simulink model "Lateral_control_of_HST"  (R2023b)
settings: Solver=ode45  StartTime=0.0  StopTime=100  FixedStep=0.001  RelTol=1e-3
InitFcn:
  | Parameters_and_initial_conditions;
values from neighbouring files (symbols this model uses):
  A_a = 2.119e-7    (= 2.119e-07)    [Parameters_and_initial_conditions.m]
  A_v = 4.032e-7    (= 4.032e-07)    [Parameters_and_initial_conditions.m]
  b = 0.7465    [Parameters_and_initial_conditions.m]
  c_px = 0    [Parameters_and_initial_conditions.m]
  c_py = 0    [Parameters_and_initial_conditions.m]
  c_pz = 1.5e4    (= 15000)    [Parameters_and_initial_conditions.m]
  c_sx = 0    [Parameters_and_initial_conditions.m]
  c_sy = 2e4    (= 20000)    [Parameters_and_initial_conditions.m]
  c_sz = 8e4    (= 80000)    [Parameters_and_initial_conditions.m]
  d_p = 1    [Parameters_and_initial_conditions.m]
  d_s = 1    [Parameters_and_initial_conditions.m]
  f_11 = 1.12e7    (= 11200000)    [Parameters_and_initial_conditions.m]
  f_22 = 9.98e6    (= 9980000)    [Parameters_and_initial_conditions.m]
  h_cs = 0.98    [Parameters_and_initial_conditions.m]
  h_ts = 0.0945    [Parameters_and_initial_conditions.m]
  h_tw = 0.1745    [Parameters_and_initial_conditions.m]
  J_cx = 89396    [Parameters_and_initial_conditions.m]
  J_cz = 2485756    [Parameters_and_initial_conditions.m]
  J_tx = 2650    [Parameters_and_initial_conditions.m]
  J_tz = 3000    [Parameters_and_initial_conditions.m]
  J_wz = 1200    [Parameters_and_initial_conditions.m]
  k11 = 1.88e7    (= 18800000)    [Parameters_and_initial_conditions.m]
  k12 = 5.807e5    (= 580700)    [Parameters_and_initial_conditions.m]
  k13 = 3.68e6    (= 3680000)    [Parameters_and_initial_conditions.m]
  k14 = 2.64e1    (= 26.4)    [Parameters_and_initial_conditions.m]
  k21 = 1.88e7    (= 18800000)    [Parameters_and_initial_conditions.m]
  k22 = 5.807e5    (= 580700)    [Parameters_and_initial_conditions.m]
  k23 = 3.68e6    (= 3680000)    [Parameters_and_initial_conditions.m]
  k24 = 2.64e1    (= 26.4)    [Parameters_and_initial_conditions.m]
  K_gpsi = -7834    [Parameters_and_initial_conditions.m]
  K_gy = 5014    [Parameters_and_initial_conditions.m]
  k_px = 1.45e7    (= 14500000)    [Parameters_and_initial_conditions.m]
  k_py = 7.5e6    (= 7500000)    [Parameters_and_initial_conditions.m]
  k_pz = 6.65e5    (= 665000)    [Parameters_and_initial_conditions.m]
  k_sx = 2.08e5    (= 208000)    [Parameters_and_initial_conditions.m]
  k_sy = 2.08e5    (= 208000)    [Parameters_and_initial_conditions.m]
  k_sz = 3.5e5    (= 350000)    [Parameters_and_initial_conditions.m]
  kd = 1    [Parameters_and_initial_conditions.m]
  kp = 3    [Parameters_and_initial_conditions.m]
  l = 9    [Parameters_and_initial_conditions.m]
  l_t = 1.25    [Parameters_and_initial_conditions.m]
  Lambda_a = 6.125e-7    (= 6.125e-07)    [Parameters_and_initial_conditions.m]
  lambda_e = 0.05    [Parameters_and_initial_conditions.m]
  Lambda_v = 1.08e-6    (= 1.08e-06)    [Parameters_and_initial_conditions.m]
  m_c = 40000    [Parameters_and_initial_conditions.m]
  m_t = 2280    [Parameters_and_initial_conditions.m]
  m_w = 1650    [Parameters_and_initial_conditions.m]
  Omega_c = 0.8246    [Parameters_and_initial_conditions.m]
  Omega_r = 0.0206    [Parameters_and_initial_conditions.m]
  Omega_s = 0.438    [Parameters_and_initial_conditions.m]
  psi_c_dot_initial = 0    [Parameters_and_initial_conditions.m]
  psi_c_initial = 0    [Parameters_and_initial_conditions.m]
  psi_t1_dot_initial = 0    [Parameters_and_initial_conditions.m]
  psi_t1_initial = 0    [Parameters_and_initial_conditions.m]
  psi_t2_dot_initial = 0    [Parameters_and_initial_conditions.m]
  psi_t2_initial = 0    [Parameters_and_initial_conditions.m]
  psi_w1_dot_initial = 0    [Parameters_and_initial_conditions.m]
  psi_w1_initial = 0    [Parameters_and_initial_conditions.m]
  psi_w2_dot_initial = 0    [Parameters_and_initial_conditions.m]
  psi_w2_initial = 0    [Parameters_and_initial_conditions.m]
  psi_w3_dot_initial = 0    [Parameters_and_initial_conditions.m]
  psi_w3_initial = 0    [Parameters_and_initial_conditions.m]
  psi_w4_dot_initial = 0    [Parameters_and_initial_conditions.m]
  psi_w4_initial = 0    [Parameters_and_initial_conditions.m]
  r_0 = 0.4575    [Parameters_and_initial_conditions.m]
  sigma = 0.05    [Parameters_and_initial_conditions.m]
  T1 = 0.15    [Parameters_and_initial_conditions.m]
  T2 = 0.04    [Parameters_and_initial_conditions.m]
  Tff = 0.1*tau    (= 0.3)    [Parameters_and_initial_conditions.m]
  Tff2 = 0.2*tau    (= 0.6)    [Parameters_and_initial_conditions.m]
  theta_c_dot_initial = 0    [Parameters_and_initial_conditions.m]
  theta_c_initial = 0    [Parameters_and_initial_conditions.m]
  theta_t1_dot_initial = 0    [Parameters_and_initial_conditions.m]
  theta_t1_initial = 0    [Parameters_and_initial_conditions.m]
  theta_t2_dot_initial = 0    [Parameters_and_initial_conditions.m]
  theta_t2_initial = 0    [Parameters_and_initial_conditions.m]
  Tnn = 0.5*tau    (= 1.5)    [Parameters_and_initial_conditions.m]
  Tnn2 = 1*tau    (= 3)    [Parameters_and_initial_conditions.m]
  V = 75    [Parameters_and_initial_conditions.m]
  y_c_dot_initial = 0    [Parameters_and_initial_conditions.m]
  y_c_initial = 0    [Parameters_and_initial_conditions.m]
  y_t1_dot_initial = 0    [Parameters_and_initial_conditions.m]
  y_t1_initial = 0    [Parameters_and_initial_conditions.m]
  y_t2_dot_initial = 0    [Parameters_and_initial_conditions.m]
  y_t2_initial = 0    [Parameters_and_initial_conditions.m]
  y_w1_dot_initial = 0    [Parameters_and_initial_conditions.m]
  y_w1_initial = 0    [Parameters_and_initial_conditions.m]
  y_w2_dot_initial = 0    [Parameters_and_initial_conditions.m]
  y_w2_initial = 0    [Parameters_and_initial_conditions.m]
  y_w3_dot_initial = 0    [Parameters_and_initial_conditions.m]
  y_w3_initial = 0    [Parameters_and_initial_conditions.m]
  y_w4_dot_initial = 0    [Parameters_and_initial_conditions.m]
  y_w4_initial = 0    [Parameters_and_initial_conditions.m]
libraries: simulink x6, dspsrcs4 x1
(part 2 of 2)

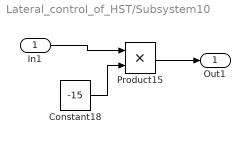
== system Lateral_control_of_HST/Subsystem10 ==
  In1 : Inport
  Constant18 : Constant  Value=-15
  Product15 : Product
  Out1 : Outport
  wires:
  Constant18/1 -> Product15/2
  In1/1 -> Product15/1
  Product15/1 -> Out1/1

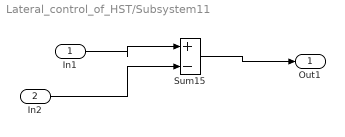
== system Lateral_control_of_HST/Subsystem11 ==
  In1 : Inport
  In2 : Inport  Port=2
  Sum15 : Sum  Inputs=|+-
  Out1 : Outport
  wires:
  In2/1 -> Sum15/2
  In1/1 -> Sum15/1
  Sum15/1 -> Out1/1

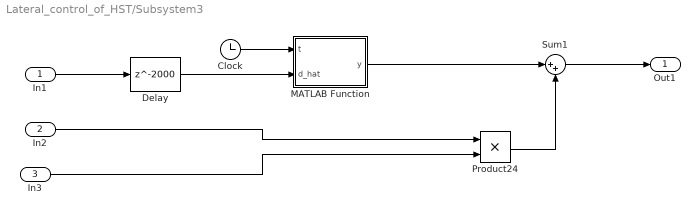
== system Lateral_control_of_HST/Subsystem3 ==
  In1 : Inport
  In2 : Inport  Port=2
  In3 : Inport  Port=3
  Clock : Clock
  Delay : Delay  DelayLength=2000
  MATLAB Function : MATLAB Function  TreatAsAtomicUnit=on
  Product24 : Product
  Sum1 : Sum  Inputs=|++
  Out1 : Outport
  wires:
  Clock/1 -> MATLAB Function/1(t)
  Product24/1 -> Sum1/2
  Sum1/1 -> Out1/1
  In2/1 -> Product24/1
  MATLAB Function/1(y) -> Sum1/1
  Delay/1 -> MATLAB Function/2(d_hat)
  In1/1 -> Delay/1
  In3/1 -> Product24/2

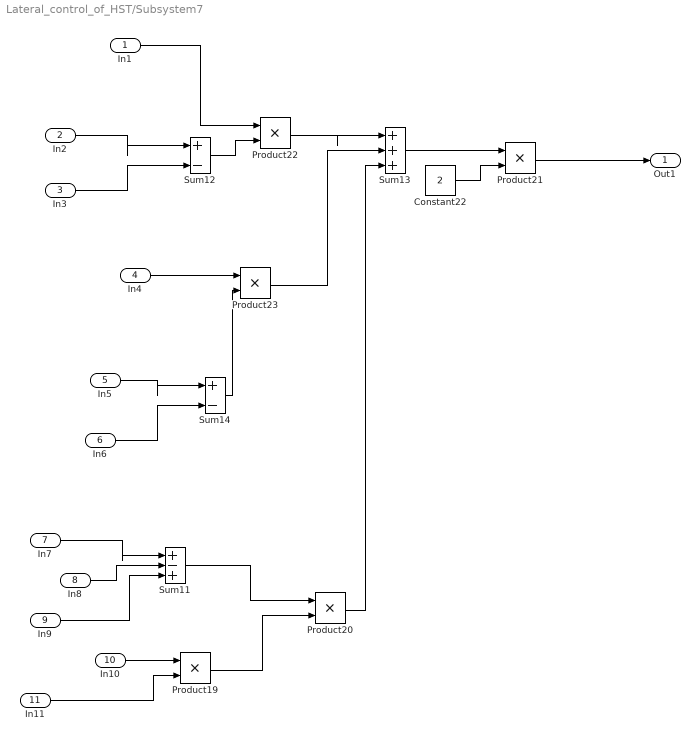
== system Lateral_control_of_HST/Subsystem7 ==
  In1 : Inport
  In2 : Inport  Port=2
  In3 : Inport  Port=3
  In4 : Inport  Port=4
  In5 : Inport  Port=5
  In6 : Inport  Port=6
  In7 : Inport  Port=7
  In8 : Inport  Port=8
  In9 : Inport  Port=9
  In10 : Inport  Port=10
  In11 : Inport  Port=11
  Constant22 : Constant  Value=2
  Product{19..23} (5 alike) : Product
  Sum11 : Sum  Inputs=|+-+
  Sum12 : Sum  Inputs=|+-
  Sum13 : Sum  Inputs=|+++
  Sum14 : Sum  Inputs=|+-
  Out1 : Outport
  wires:
  Product22/1 -> Sum13/1
  In5/1 -> Sum14/1
  Sum13/1 -> Product21/1
  In6/1 -> Sum14/2
  Sum11/1 -> Product20/1
  Product19/1 -> Product20/2
  Sum14/1 -> Product23/2
  In7/1 -> Sum11/1
  Product23/1 -> Sum13/2
  Sum12/1 -> Product22/2
  In2/1 -> Sum12/1
  Product20/1 -> Sum13/3
  Constant22/1 -> Product21/2
  In10/1 -> Product19/1
  In9/1 -> Sum11/3
  In4/1 -> Product23/1
  In3/1 -> Sum12/2
  In1/1 -> Product22/1
  Product21/1 -> Out1/1
  In11/1 -> Product19/2
  In8/1 -> Sum11/2

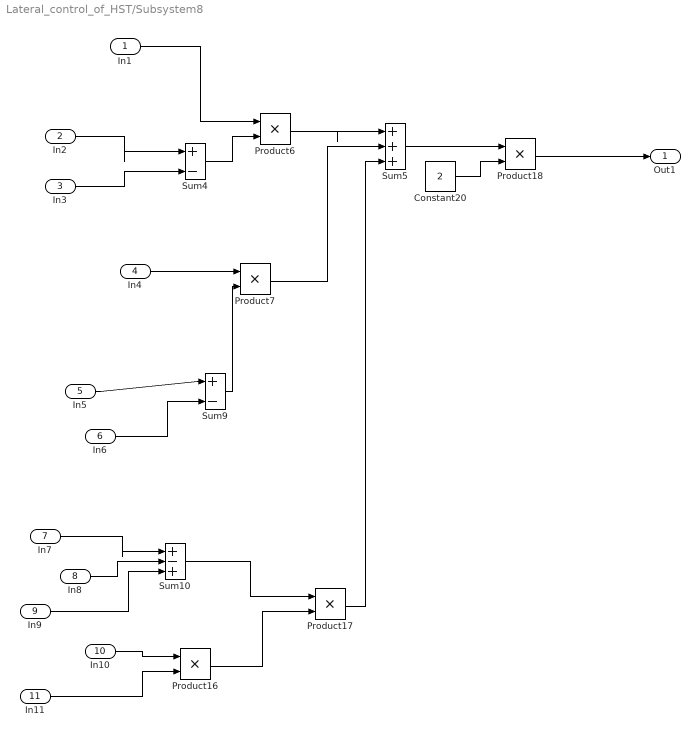
== system Lateral_control_of_HST/Subsystem8 ==
  In1 : Inport
  In2 : Inport  Port=2
  In3 : Inport  Port=3
  In4 : Inport  Port=4
  In5 : Inport  Port=5
  In6 : Inport  Port=6
  In7 : Inport  Port=7
  In8 : Inport  Port=8
  In9 : Inport  Port=9
  In10 : Inport  Port=10
  In11 : Inport  Port=11
  Constant20 : Constant  Value=2
  Product{6..7,16..18} (5 alike) : Product
  Sum10 : Sum  Inputs=|+-+
  Sum4 : Sum  Inputs=|+-
  Sum5 : Sum  Inputs=|+++
  Sum9 : Sum  Inputs=|+-
  Out1 : Outport
  wires:
  Constant20/1 -> Product18/2
  Product6/1 -> Sum5/1
  Sum9/1 -> Product7/2
  Product17/1 -> Sum5/3
  Sum4/1 -> Product6/2
  In6/1 -> Sum9/2
  Product16/1 -> Product17/2
  Sum5/1 -> Product18/1
  In9/1 -> Sum10/3
  Product7/1 -> Sum5/2
  In1/1 -> Product6/1
  Sum10/1 -> Product17/1
  Product18/1 -> Out1/1
  In8/1 -> Sum10/2
  In4/1 -> Product7/1
  In5/1 -> Sum9/1
  In7/1 -> Sum10/1
  In3/1 -> Sum4/2
  In2/1 -> Sum4/1
  In11/1 -> Product16/2
  In10/1 -> Product16/1

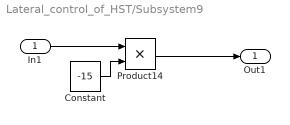
== system Lateral_control_of_HST/Subsystem9 ==
  In1 : Inport
  Constant : Constant  Value=-15
  Product14 : Product
  Out1 : Outport
  wires:
  Constant/1 -> Product14/2
  In1/1 -> Product14/1
  Product14/1 -> Out1/1

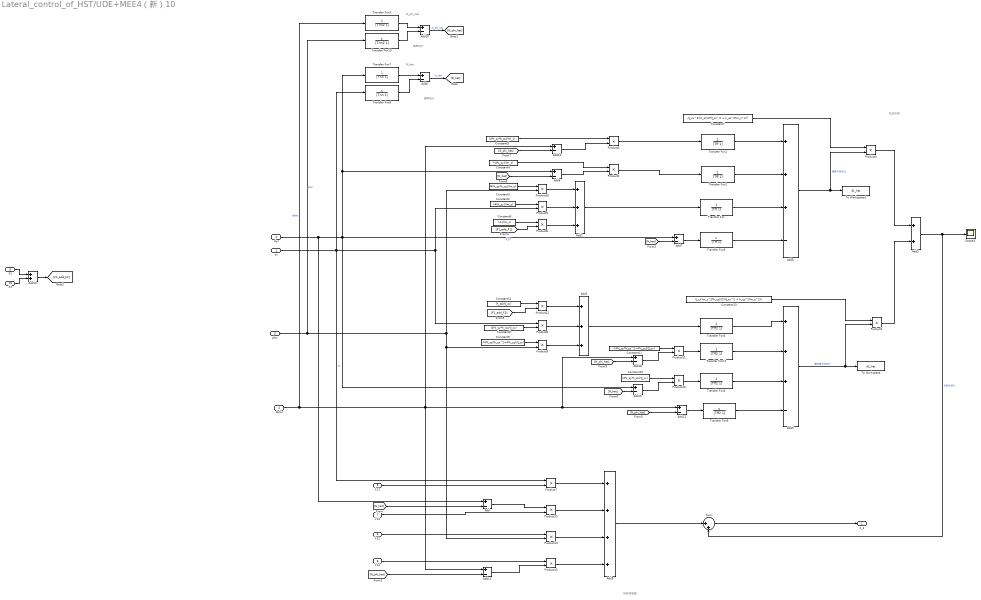
== system Lateral_control_of_HST/UDE+MEE4（新）10 ==
  note: 扰动补偿
  note: 噪声估计
  note: 标称控制器
  note: N_phi_hat
  note: N_hat
  note: 噪声估计
  yc : Inport
  dyc : Inport  Port=2
  phic : Inport  Port=3
  dphic : Inport  Port=4
  k11 : Inport  Port=5
  k12 : Inport  Port=6
  k13 : Inport  Port=7
  k14 : Inport  Port=8
  F1 : Inport  Port=9
  F2 : Inport  Port=10
  Add{,4,6..7,10..12,14..16} (10 alike) : Sum  Inputs=+-
  Add1 : Sum  Inputs=+++
  Add13 : Sum
  Add2 : Sum  Inputs=+++
  Add3 : Sum
  Add5 : Sum  Inputs=+++-
  Add8 : Sum  Inputs=+++-
  Add9 : Sum  Inputs=++++
  Constant10 : Constant  Value=(4*c_sy*h_cs)/(J_cx)
  Constant11 : Constant  Value=-(4*c_sy*h_cs^2+4*c_sz)/(J_cx)
  Constant12 : Constant  Value=(h_cs)/(J_cx)
  Constant13 : Constant  Value=(J_cx*m_c^2*h_cs)/(2*(J_cx^2 + h_cs^2*m_c^2))
  Constant2 : Constant  Value=(-4*k_sy)/(m_c)
  Constant3 : Constant  Value=(4*k_sy*h_cs)/(m_c)
  Constant4 : Constant  Value=(-4*c_sy)/(m_c)
  Constant5 : Constant  Value=(4*c_sy*h_cs)/(m_c)
  Constant6 : Constant  Value=(-1)/(m_c)
  Constant7 : Constant  Value=-(J_cx^2*m_c)/(2*(J_cx^2 + h_cs^2*m_c^2))
  Constant8 : Constant  Value=(4*k_sy*h_cs)/(J_cx)  VectorParams1D=off
  Constant9 : Constant  Value=-(4*k_sy*h_cs^2+4*k_sz)/(J_cx)
  Product{1..16} (16 alike) : Product
  Scope3 : Scope
  Sum : Sum  Inputs=|++
  To Workspace : ToWorkspace  VariableName=d2_hat  SaveFormat=Timeseries  SampleTime=-1
  To Workspace1 : ToWorkspace  VariableName=d1_hat  SaveFormat=Timeseries  SampleTime=-1
  Transfer Fcn : TransferFcn  Denominator=[Tff 1]
  Transfer Fcn1 : TransferFcn  Denominator=[Tff 1]
  Transfer Fcn10 : TransferFcn  Numerator=[1 0]  Denominator=[Tnn2 1]
  Transfer Fcn11 : TransferFcn  Denominator=[Tff2 1]
  Transfer Fcn2 : TransferFcn  Denominator=[Tff 1]
  Transfer Fcn3 : TransferFcn  Denominator=[Tnn2 1]
  Transfer Fcn4 : TransferFcn  Denominator=[Tff2 1]
  Transfer Fcn5 : TransferFcn  Denominator=[Tff2 1]
  Transfer Fcn6 : TransferFcn  Numerator=[1 0]  Denominator=[Tff 1]
  Transfer Fcn7 : TransferFcn  Denominator=[Tnn 1]
  Transfer Fcn8 : TransferFcn  Numerator=[1 0]  Denominator=[Tnn 1]
  Transfer Fcn9 : TransferFcn  Numerator=[1 0]  Denominator=[Tff2 1]
  F_1 : Outport
  wires:
  yc/1 -> Product5/2, Product8/1, Transfer Fcn8/1, Product7/1  "yc"
  dyc/1 -> Add7/1, Add15/1, Add4/1, Transfer Fcn7/1, Add/1  "d_yc"
  dphic/1 -> Add11/1, Add16/1, Add14/1, Add12/1, Transfer Fcn3/1  "dphic"
  k11/1 -> Product7/2
  k12/1 -> Product14/1
  k13/1 -> Product13/2
  k14/1 -> Product15/1
  Constant6/1 -> Product6/1
  Constant8/1 -> Product8/2
  Constant9/1 -> Product9/1
  Constant12/1 -> Product12/1
  Add3/1 -> Scope3/1, Sum/2  "总扰动估计"
  Sum/1 -> F_1/1
  Add1/1 -> Transfer Fcn/1
  Constant7/1 -> Product3/1
  Product3/1 -> Add3/1
  Constant2/1 -> Product5/1
  Constant3/1 -> Product16/1
  Product5/1 -> Add1/2
  Product6/1 -> Add1/3
  Constant4/1 -> Product2/1
  Product2/1 -> Transfer Fcn2/1
  Transfer Fcn7/1 -> Add6/1
  Transfer Fcn8/1 -> Add6/2
  Add6/1 -> [N_hat]  "N_hat"
  Add7/1 -> Transfer Fcn6/1
  Add8/1 -> To Workspace1/1, Product3/2  "横移方向估计"
  Product12/1 -> Add2/1
  Product9/1 -> Add2/3
  Constant10/1 -> Product10/1
  Product10/1 -> Transfer Fcn4/1
  Add2/1 -> Transfer Fcn5/1
  Transfer Fcn5/1 -> Add5/1
  Constant13/1 -> Product1/1
  Add5/1 -> To Workspace/1, Product1/2  "翻滚角方向估计"
  Product1/1 -> Add3/2
  Product7/1 -> Add9/1
  [N_hat] -> Add/2
  Add/1 -> Product13/1
  Product13/1 -> Add9/2
  phic/1 -> Transfer Fcn10/1, Product14/2, Product9/2, Product16/2  "phic"
  Product14/1 -> Add9/3
  Add12/1 -> Product15/2
  Product15/1 -> Add9/4
  Add9/1 -> Sum/1
  Product16/1 -> Add1/1
  Product4/1 -> Transfer Fcn1/1
  Constant5/1 -> Product4/1
  Transfer Fcn1/1 -> Add8/1
  Transfer Fcn2/1 -> Add8/2
  Transfer Fcn6/1 -> Add8/4
  Transfer Fcn/1 -> Add8/3
  Transfer Fcn3/1 -> Add10/1
  Add10/1 -> [N_phi_hat]  "N_phi_hat"
  Transfer Fcn10/1 -> Add10/2
  Product11/1 -> Transfer Fcn11/1
  Transfer Fcn9/1 -> Add5/4
  Add11/1 -> Transfer Fcn9/1
  Product8/1 -> Add2/2
  [N_phi_hat] -> Add12/2
  [N_hat] -> Add7/2
  [N_phi_hat] -> Add11/2
  Transfer Fcn4/1 -> Add5/3
  Transfer Fcn11/1 -> Add5/2
  F1/1 -> Add13/1
  F2/1 -> Add13/2
  Add13/1 -> [F1_add_F2]
  [F1_add_F2] -> Product6/2
  [F1_add_F2] -> Product12/2
  Constant11/1 -> Product11/1
  Add4/1 -> Product2/2
  [N_hat] -> Add4/2
  Add14/1 -> Product4/2
  [N_phi_hat] -> Add14/2
  Add15/1 -> Product10/2
  [N_hat] -> Add15/2
  Add16/1 -> Product11/2
  [N_phi_hat] -> Add16/2

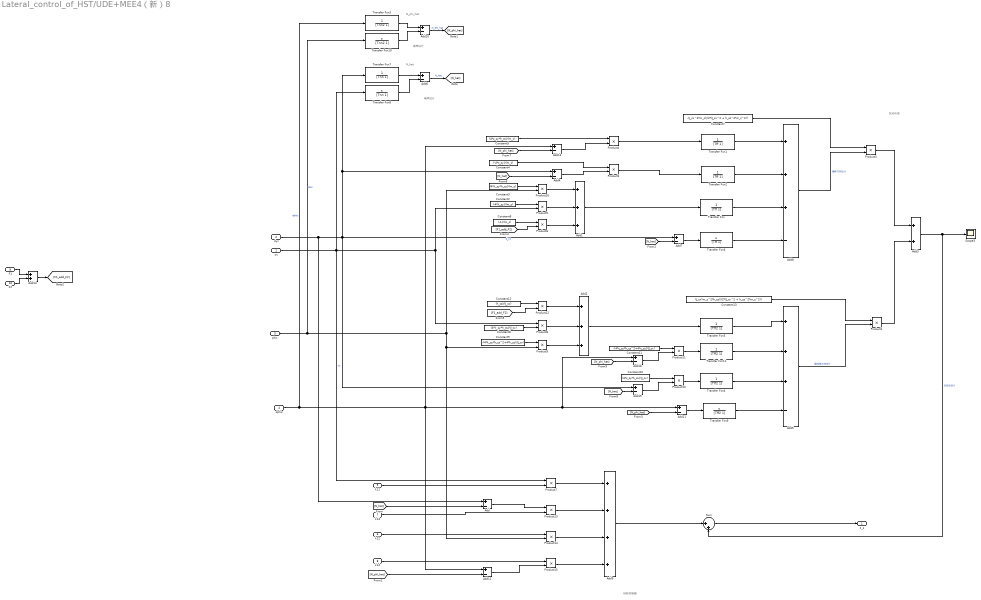
== system Lateral_control_of_HST/UDE+MEE4（新）8 ==
  note: 扰动补偿
  note: 噪声估计
  note: 标称控制器
  note: N_phi_hat
  note: N_hat
  note: 噪声估计
  yc : Inport
  dyc : Inport  Port=2
  phic : Inport  Port=3
  dphic : Inport  Port=4
  k11 : Inport  Port=5
  k12 : Inport  Port=6
  k13 : Inport  Port=7
  k14 : Inport  Port=8
  F1 : Inport  Port=9
  F2 : Inport  Port=10
  Add{,4,6..7,10..12,14..16} (10 alike) : Sum  Inputs=+-
  Add1 : Sum  Inputs=+++
  Add13 : Sum
  Add2 : Sum  Inputs=+++
  Add3 : Sum
  Add5 : Sum  Inputs=+++-
  Add8 : Sum  Inputs=+++-
  Add9 : Sum  Inputs=++++
  Constant10 : Constant  Value=(4*c_sy*h_cs)/(J_cx)
  Constant11 : Constant  Value=-(4*c_sy*h_cs^2+4*c_sz)/(J_cx)
  Constant12 : Constant  Value=(h_cs)/(J_cx)
  Constant13 : Constant  Value=(J_cx*m_c^2*h_cs)/(2*(J_cx^2 + h_cs^2*m_c^2))
  Constant2 : Constant  Value=(-4*k_sy)/(m_c)
  Constant3 : Constant  Value=(4*k_sy*h_cs)/(m_c)
  Constant4 : Constant  Value=(-4*c_sy)/(m_c)
  Constant5 : Constant  Value=(4*c_sy*h_cs)/(m_c)
  Constant6 : Constant  Value=(-1)/(m_c)
  Constant7 : Constant  Value=-(J_cx^2*m_c)/(2*(J_cx^2 + h_cs^2*m_c^2))
  Constant8 : Constant  Value=(4*k_sy*h_cs)/(J_cx)  VectorParams1D=off
  Constant9 : Constant  Value=-(4*k_sy*h_cs^2+4*k_sz)/(J_cx)
  Product{1..16} (16 alike) : Product
  Scope3 : Scope
  Sum : Sum  Inputs=|++
  Transfer Fcn : TransferFcn  Denominator=[Tff 1]
  Transfer Fcn1 : TransferFcn  Denominator=[Tff 1]
  Transfer Fcn10 : TransferFcn  Numerator=[1 0]  Denominator=[Tnn2 1]
  Transfer Fcn11 : TransferFcn  Denominator=[Tff2 1]
  Transfer Fcn2 : TransferFcn  Denominator=[Tff 1]
  Transfer Fcn3 : TransferFcn  Denominator=[Tnn2 1]
  Transfer Fcn4 : TransferFcn  Denominator=[Tff2 1]
  Transfer Fcn5 : TransferFcn  Denominator=[Tff2 1]
  Transfer Fcn6 : TransferFcn  Numerator=[1 0]  Denominator=[Tff 1]
  Transfer Fcn7 : TransferFcn  Denominator=[Tnn 1]
  Transfer Fcn8 : TransferFcn  Numerator=[1 0]  Denominator=[Tnn 1]
  Transfer Fcn9 : TransferFcn  Numerator=[1 0]  Denominator=[Tff2 1]
  F_1 : Outport
  wires:
  yc/1 -> Product5/2, Product8/1, Transfer Fcn8/1, Product7/1  "yc"
  dyc/1 -> Add7/1, Add15/1, Add4/1, Transfer Fcn7/1, Add/1  "d_yc"
  dphic/1 -> Add11/1, Add16/1, Add14/1, Add12/1, Transfer Fcn3/1  "dphic"
  k11/1 -> Product7/2
  k12/1 -> Product14/1
  k13/1 -> Product13/2
  k14/1 -> Product15/1
  Constant6/1 -> Product6/1
  Constant8/1 -> Product8/2
  Constant9/1 -> Product9/1
  Constant12/1 -> Product12/1
  Add3/1 -> Scope3/1, Sum/2  "总扰动估计"
  Sum/1 -> F_1/1
  Add1/1 -> Transfer Fcn/1
  Constant7/1 -> Product3/1
  Product3/1 -> Add3/1
  Constant2/1 -> Product5/1
  Constant3/1 -> Product16/1
  Product5/1 -> Add1/2
  Product6/1 -> Add1/3
  Constant4/1 -> Product2/1
  Product2/1 -> Transfer Fcn2/1
  Transfer Fcn7/1 -> Add6/1
  Transfer Fcn8/1 -> Add6/2
  Add6/1 -> [N_hat]  "N_hat"
  Add7/1 -> Transfer Fcn6/1
  Add8/1 -> Product3/2  "横移方向估计"
  Product12/1 -> Add2/1
  Product9/1 -> Add2/3
  Constant10/1 -> Product10/1
  Product10/1 -> Transfer Fcn4/1
  Add2/1 -> Transfer Fcn5/1
  Transfer Fcn5/1 -> Add5/1
  Constant13/1 -> Product1/1
  Add5/1 -> Product1/2  "翻滚角方向估计"
  Product1/1 -> Add3/2
  Product7/1 -> Add9/1
  [N_hat] -> Add/2
  Add/1 -> Product13/1
  Product13/1 -> Add9/2
  phic/1 -> Transfer Fcn10/1, Product14/2, Product9/2, Product16/2  "phic"
  Product14/1 -> Add9/3
  Add12/1 -> Product15/2
  Product15/1 -> Add9/4
  Add9/1 -> Sum/1
  Product16/1 -> Add1/1
  Product4/1 -> Transfer Fcn1/1
  Constant5/1 -> Product4/1
  Transfer Fcn1/1 -> Add8/1
  Transfer Fcn2/1 -> Add8/2
  Transfer Fcn6/1 -> Add8/4
  Transfer Fcn/1 -> Add8/3
  Transfer Fcn3/1 -> Add10/1
  Add10/1 -> [N_phi_hat]  "N_phi_hat"
  Transfer Fcn10/1 -> Add10/2
  Product11/1 -> Transfer Fcn11/1
  Transfer Fcn9/1 -> Add5/4
  Add11/1 -> Transfer Fcn9/1
  Product8/1 -> Add2/2
  [N_phi_hat] -> Add12/2
  [N_hat] -> Add7/2
  [N_phi_hat] -> Add11/2
  Transfer Fcn4/1 -> Add5/3
  Transfer Fcn11/1 -> Add5/2
  F1/1 -> Add13/1
  F2/1 -> Add13/2
  Add13/1 -> [F1_add_F2]
  [F1_add_F2] -> Product6/2
  [F1_add_F2] -> Product12/2
  Constant11/1 -> Product11/1
  Add4/1 -> Product2/2
  [N_hat] -> Add4/2
  Add14/1 -> Product4/2
  [N_phi_hat] -> Add14/2
  Add15/1 -> Product10/2
  [N_hat] -> Add15/2
  Add16/1 -> Product11/2
  [N_phi_hat] -> Add16/2

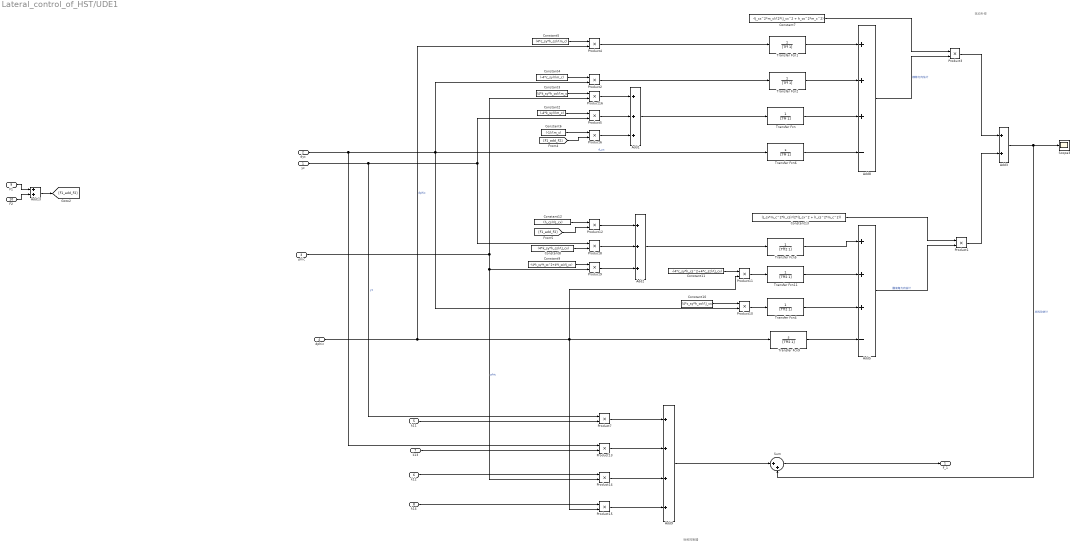
== system Lateral_control_of_HST/UDE1 ==
  note: 扰动补偿
  note: 标称控制器
  yc : Inport
  dyc : Inport  Port=2
  phic : Inport  Port=3
  dphic : Inport  Port=4
  k11 : Inport  Port=5
  k12 : Inport  Port=6
  k13 : Inport  Port=7
  k14 : Inport  Port=8
  F1 : Inport  Port=9
  F2 : Inport  Port=10
  Add1 : Sum  Inputs=+++
  Add13 : Sum
  Add2 : Sum  Inputs=+++
  Add3 : Sum
  Add5 : Sum  Inputs=+++-
  Add8 : Sum  Inputs=+++-
  Add9 : Sum  Inputs=++++
  Constant10 : Constant  Value=(4*c_sy*h_cs)/(J_cx)
  Constant11 : Constant  Value=-(4*c_sy*h_cs^2+4*c_sz)/(J_cx)
  Constant12 : Constant  Value=(h_cs)/(J_cx)
  Constant13 : Constant  Value=(J_cx*m_c^2*h_cs)/(2*(J_cx^2 + h_cs^2*m_c^2))
  Constant2 : Constant  Value=(-4*k_sy)/(m_c)
  Constant3 : Constant  Value=(4*k_sy*h_cs)/(m_c)
  Constant4 : Constant  Value=(-4*c_sy)/(m_c)
  Constant5 : Constant  Value=(4*c_sy*h_cs)/(m_c)
  Constant6 : Constant  Value=(-1)/(m_c)
  Constant7 : Constant  Value=-(J_cx^2*m_c)/(2*(J_cx^2 + h_cs^2*m_c^2))
  Constant8 : Constant  Value=(4*k_sy*h_cs)/(J_cx)  VectorParams1D=off
  Constant9 : Constant  Value=-(4*k_sy*h_cs^2+4*k_sz)/(J_cx)
  Product{1..16} (16 alike) : Product
  Scope3 : Scope
  Sum : Sum  Inputs=|++
  Transfer Fcn : TransferFcn  Denominator=[Tff 1]
  Transfer Fcn1 : TransferFcn  Denominator=[Tff 1]
  Transfer Fcn11 : TransferFcn  Denominator=[Tff2 1]
  Transfer Fcn2 : TransferFcn  Denominator=[Tff 1]
  Transfer Fcn4 : TransferFcn  Denominator=[Tff2 1]
  Transfer Fcn5 : TransferFcn  Denominator=[Tff2 1]
  Transfer Fcn6 : TransferFcn  Numerator=[1 0]  Denominator=[Tff 1]
  Transfer Fcn9 : TransferFcn  Numerator=[1 0]  Denominator=[Tff2 1]
  F_1 : Outport
  wires:
  yc/1 -> Product5/2, Product8/1, Product7/1  "yc"
  dyc/1 -> Product13/1, Product2/2, Product10/2, Transfer Fcn6/1  "d_yc"
  dphic/1 -> Transfer Fcn9/1, Product11/2, Product15/2, Product4/2  "dphic"
  k11/1 -> Product7/2
  k12/1 -> Product14/1
  k13/1 -> Product13/2
  k14/1 -> Product15/1
  Constant6/1 -> Product6/1
  Constant8/1 -> Product8/2
  Constant9/1 -> Product9/1
  Constant12/1 -> Product12/1
  Add3/1 -> Scope3/1, Sum/2  "总扰动估计"
  Sum/1 -> F_1/1
  Add1/1 -> Transfer Fcn/1
  Constant7/1 -> Product3/1
  Product3/1 -> Add3/1
  Constant2/1 -> Product5/1
  Constant3/1 -> Product16/1
  Product5/1 -> Add1/2
  Product6/1 -> Add1/3
  Constant4/1 -> Product2/1
  Product2/1 -> Transfer Fcn2/1
  Add8/1 -> Product3/2  "横移方向估计"
  Product12/1 -> Add2/1
  Product9/1 -> Add2/3
  Constant10/1 -> Product10/1
  Product10/1 -> Transfer Fcn4/1
  Add2/1 -> Transfer Fcn5/1
  Transfer Fcn5/1 -> Add5/1
  Constant13/1 -> Product1/1
  Add5/1 -> Product1/2  "翻滚角方向估计"
  Product1/1 -> Add3/2
  Product7/1 -> Add9/1
  Product13/1 -> Add9/2
  phic/1 -> Product16/2, Product14/2, Product9/2  "phic"
  Product14/1 -> Add9/3
  Product15/1 -> Add9/4
  Add9/1 -> Sum/1
  Product16/1 -> Add1/1
  Product4/1 -> Transfer Fcn1/1
  Constant5/1 -> Product4/1
  Transfer Fcn1/1 -> Add8/1
  Transfer Fcn2/1 -> Add8/2
  Transfer Fcn6/1 -> Add8/4
  Transfer Fcn/1 -> Add8/3
  Product11/1 -> Transfer Fcn11/1
  Transfer Fcn9/1 -> Add5/4
  Product8/1 -> Add2/2
  Transfer Fcn4/1 -> Add5/3
  Transfer Fcn11/1 -> Add5/2
  F1/1 -> Add13/1
  F2/1 -> Add13/2
  Add13/1 -> [F1_add_F2]
  [F1_add_F2] -> Product6/2
  [F1_add_F2] -> Product12/2
  Constant11/1 -> Product11/1

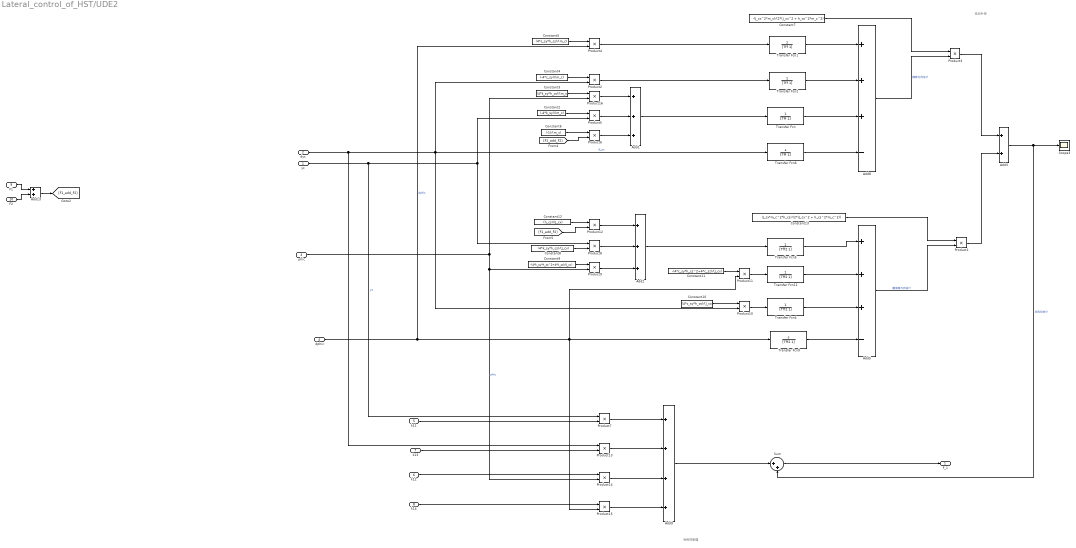
== system Lateral_control_of_HST/UDE2 ==
  note: 扰动补偿
  note: 标称控制器
  yc : Inport
  dyc : Inport  Port=2
  phic : Inport  Port=3
  dphic : Inport  Port=4
  k11 : Inport  Port=5
  k12 : Inport  Port=6
  k13 : Inport  Port=7
  k14 : Inport  Port=8
  F1 : Inport  Port=9
  F2 : Inport  Port=10
  Add1 : Sum  Inputs=+++
  Add13 : Sum
  Add2 : Sum  Inputs=+++
  Add3 : Sum
  Add5 : Sum  Inputs=+++-
  Add8 : Sum  Inputs=+++-
  Add9 : Sum  Inputs=++++
  Constant10 : Constant  Value=(4*c_sy*h_cs)/(J_cx)
  Constant11 : Constant  Value=-(4*c_sy*h_cs^2+4*c_sz)/(J_cx)
  Constant12 : Constant  Value=(h_cs)/(J_cx)
  Constant13 : Constant  Value=(J_cx*m_c^2*h_cs)/(2*(J_cx^2 + h_cs^2*m_c^2))
  Constant2 : Constant  Value=(-4*k_sy)/(m_c)
  Constant3 : Constant  Value=(4*k_sy*h_cs)/(m_c)
  Constant4 : Constant  Value=(-4*c_sy)/(m_c)
  Constant5 : Constant  Value=(4*c_sy*h_cs)/(m_c)
  Constant6 : Constant  Value=(-1)/(m_c)
  Constant7 : Constant  Value=-(J_cx^2*m_c)/(2*(J_cx^2 + h_cs^2*m_c^2))
  Constant8 : Constant  Value=(4*k_sy*h_cs)/(J_cx)  VectorParams1D=off
  Constant9 : Constant  Value=-(4*k_sy*h_cs^2+4*k_sz)/(J_cx)
  Product{1..16} (16 alike) : Product
  Scope3 : Scope
  Sum : Sum  Inputs=|++
  Transfer Fcn : TransferFcn  Denominator=[Tff 1]
  Transfer Fcn1 : TransferFcn  Denominator=[Tff 1]
  Transfer Fcn11 : TransferFcn  Denominator=[Tff2 1]
  Transfer Fcn2 : TransferFcn  Denominator=[Tff 1]
  Transfer Fcn4 : TransferFcn  Denominator=[Tff2 1]
  Transfer Fcn5 : TransferFcn  Denominator=[Tff2 1]
  Transfer Fcn6 : TransferFcn  Numerator=[1 0]  Denominator=[Tff 1]
  Transfer Fcn9 : TransferFcn  Numerator=[1 0]  Denominator=[Tff2 1]
  F_1 : Outport
  wires:
  yc/1 -> Product5/2, Product8/1, Product7/1  "yc"
  dyc/1 -> Product13/1, Product2/2, Product10/2, Transfer Fcn6/1  "d_yc"
  dphic/1 -> Transfer Fcn9/1, Product11/2, Product15/2, Product4/2  "dphic"
  k11/1 -> Product7/2
  k12/1 -> Product14/1
  k13/1 -> Product13/2
  k14/1 -> Product15/1
  Constant6/1 -> Product6/1
  Constant8/1 -> Product8/2
  Constant9/1 -> Product9/1
  Constant12/1 -> Product12/1
  Add3/1 -> Scope3/1, Sum/2  "总扰动估计"
  Sum/1 -> F_1/1
  Add1/1 -> Transfer Fcn/1
  Constant7/1 -> Product3/1
  Product3/1 -> Add3/1
  Constant2/1 -> Product5/1
  Constant3/1 -> Product16/1
  Product5/1 -> Add1/2
  Product6/1 -> Add1/3
  Constant4/1 -> Product2/1
  Product2/1 -> Transfer Fcn2/1
  Add8/1 -> Product3/2  "横移方向估计"
  Product12/1 -> Add2/1
  Product9/1 -> Add2/3
  Constant10/1 -> Product10/1
  Product10/1 -> Transfer Fcn4/1
  Add2/1 -> Transfer Fcn5/1
  Transfer Fcn5/1 -> Add5/1
  Constant13/1 -> Product1/1
  Add5/1 -> Product1/2  "翻滚角方向估计"
  Product1/1 -> Add3/2
  Product7/1 -> Add9/1
  Product13/1 -> Add9/2
  phic/1 -> Product16/2, Product14/2, Product9/2  "phic"
  Product14/1 -> Add9/3
  Product15/1 -> Add9/4
  Add9/1 -> Sum/1
  Product16/1 -> Add1/1
  Product4/1 -> Transfer Fcn1/1
  Constant5/1 -> Product4/1
  Transfer Fcn1/1 -> Add8/1
  Transfer Fcn2/1 -> Add8/2
  Transfer Fcn6/1 -> Add8/4
  Transfer Fcn/1 -> Add8/3
  Product11/1 -> Transfer Fcn11/1
  Transfer Fcn9/1 -> Add5/4
  Product8/1 -> Add2/2
  Transfer Fcn4/1 -> Add5/3
  Transfer Fcn11/1 -> Add5/2
  F1/1 -> Add13/1
  F2/1 -> Add13/2
  Add13/1 -> [F1_add_F2]
  [F1_add_F2] -> Product6/2
  [F1_add_F2] -> Product12/2
  Constant11/1 -> Product11/1

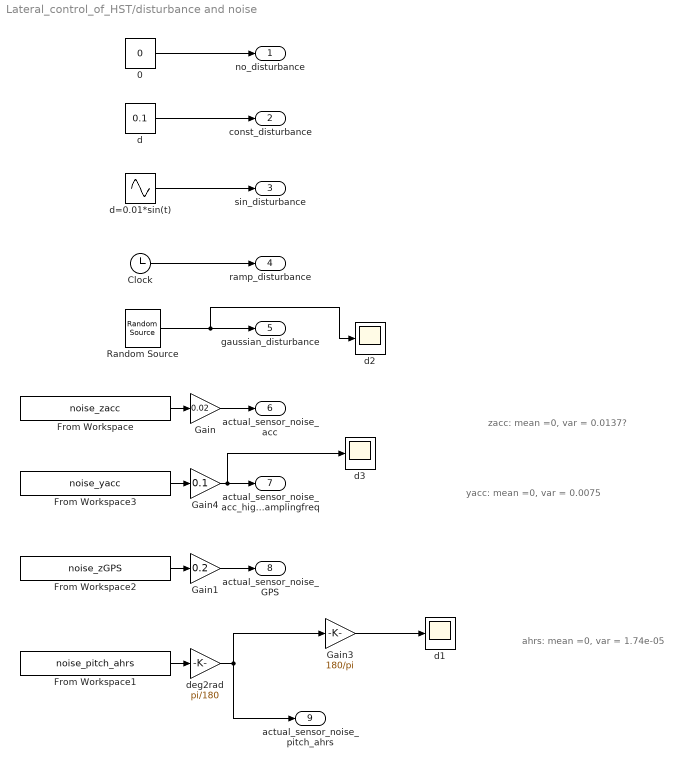
== system Lateral_control_of_HST/disturbance and noise ==
  note: ahrs: mean =0, var = 1.74e-05
  note: zacc: mean =0, var = 0.0137?
  note: yacc: mean =0, var = 0.0075
  0 : Constant  Value=0
  Clock : Clock
  From Workspace : FromWorkspace  VariableName=noise_zacc  SampleTime=-1  OutputAfterFinalValue=Setting to zero
  From Workspace1 : FromWorkspace  VariableName=noise_pitch_ahrs  SampleTime=-1  OutputAfterFinalValue=Setting to zero
  From Workspace2 : FromWorkspace  VariableName=noise_zGPS  SampleTime=-1  OutputAfterFinalValue=Setting to zero
  From Workspace3 : FromWorkspace  VariableName=noise_yacc  SampleTime=-1  OutputAfterFinalValue=Setting to zero
  Gain : Gain  Gain=0.02
  Gain1 : Gain  Gain=0.2
  Gain3 : Gain  Gain=180/pi
  Gain4 : Gain  Gain=0.1
  Random Source : dspsrcs4/Random Source  SrcType=Gaussian  NormMethod=Ziggurat  CltLength=12  MinVal=0  MaxVal=1  MeanVal=0  VarVal=0.01  RepMode=Repeatable  rawSeed=1  IsInherit=off  SampMode=Continuous  SampTime=1  SampFrame=1  DataType=Double  OutComplex=Real  OutputFrames=on
  d : Constant  Value=0.1
  d1 : Scope
  d2 : Scope
  d3 : Scope
  d=0.01*sin(t) : Sin  Amplitude=0.01  SampleTime=0
  deg2rad : Gain  Gain=pi/180
  no_disturbance : Outport  VectorParamsAs1DForOutWhenUnconnected=off
  const_disturbance : Outport  Port=2  VectorParamsAs1DForOutWhenUnconnected=off
  sin_disturbance : Outport  Port=3  VectorParamsAs1DForOutWhenUnconnected=off
  ramp_disturbance : Outport  Port=4  VectorParamsAs1DForOutWhenUnconnected=off
  gaussian_disturbance : Outport  Port=5  VectorParamsAs1DForOutWhenUnconnected=off
  actual_sensor_noise_acc : Outport  Port=6  VectorParamsAs1DForOutWhenUnconnected=off
  actual_sensor_noise_acc_highsamplingfreq : Outport  Port=7  VectorParamsAs1DForOutWhenUnconnected=off
  actual_sensor_noise_GPS : Outport  Port=8  VectorParamsAs1DForOutWhenUnconnected=off
  actual_sensor_noise_pitch_ahrs : Outport  Port=9  VectorParamsAs1DForOutWhenUnconnected=off
  wires:
  d/1 -> const_disturbance/1
  d=0.01*sin(t)/1 -> sin_disturbance/1
  Clock/1 -> ramp_disturbance/1
  From Workspace/1 -> Gain/1
  Gain/1 -> actual_sensor_noise_acc/1
  Random Source/1 -> d2/1, gaussian_disturbance/1
  From Workspace2/1 -> Gain1/1
  Gain1/1 -> actual_sensor_noise_GPS/1
  0/1 -> no_disturbance/1
  From Workspace1/1 -> deg2rad/1
  From Workspace3/1 -> Gain4/1
  Gain4/1 -> d3/1, actual_sensor_noise_acc_highsamplingfreq/1
  deg2rad/1 -> Gain3/1, actual_sensor_noise_pitch_ahrs/1
  Gain3/1 -> d1/1

== matlab function Lateral_control_of_HST/Differential equation of y_t1 ==
  data: m_t input; y_t1_ddot output; k_sy input; y_c input; l input; psi_c input; h_cs input; theta_c input; y_t1 input; h_ts input; theta_t1 input; c_sy input; y_c_dot input; psi_c_dot input; theta_c_dot input; y_t1_dot input; theta_t1_dot input; k_py input; h_tp input; y_w1 input; y_w2 input; c_py input; y_w1_dot input; y_w2_dot input; f_1 input
function y_t1_ddot = fcn(m_t,k_sy,y_c,l,psi_c,h_cs,theta_c,y_t1,h_ts,theta_t1,c_sy,y_c_dot,psi_c_dot,theta_c_dot,y_t1_dot,theta_t1_dot,k_py,h_tp,y_w1,y_w2,c_py,y_w1_dot,y_w2_dot,f_1)
y_t1_ddot = 0;
y_t1_ddot = 2*k_sy*(y_c+l*psi_c-h_cs*theta_c-y_t1-h_ts*theta_t1)+2*c_sy*(y_c_dot+l*psi_c_dot-h_cs*theta_c_dot-y_t1_dot-h_ts*theta_t1_dot)-2*k_py*(2*y_t1-2*h_tp*theta_t1-y_w1-y_w2)-2*c_py*(2*y_t1_dot-2*h_tp*theta_t1_dot-y_w1_dot-y_w2_dot)+f_1;
y_t1_ddot = y_t1_ddot/m_t;
end

== matlab function Lateral_control_of_HST/Differential equation of y_t2 ==
  data: m_t input; y_t2_ddot output; k_sy input; y_c input; l input; psi_c input; h_cs input; theta_c input; y_t2 input; h_ts input; theta_t2 input; c_sy input; y_c_dot input; psi_c_dot input; theta_c_dot input; y_t2_dot input; theta_t2_dot input; k_py input; h_tp input; y_w3 input; y_w4 input; c_py input; y_w3_dot input; y_w4_dot input; f_2 input
function y_t2_ddot = fcn(m_t,k_sy,y_c,l,psi_c,h_cs,theta_c,y_t2,h_ts,theta_t2,c_sy,y_c_dot,psi_c_dot,theta_c_dot,y_t2_dot,theta_t2_dot,k_py,h_tp,y_w3,y_w4,c_py,y_w3_dot,y_w4_dot,f_2)
y_t2_ddot = 0 ;
y_t2_ddot = 2*k_sy*(y_c-l*psi_c-h_cs*theta_c-y_t2-h_ts*theta_t2)+2*c_sy*(y_c_dot-l*psi_c_dot-h_cs*theta_c_dot-y_t2_dot-h_ts*theta_t2_dot)-2*k_py*(2*y_t2-2*h_tp*theta_t2-y_w3-y_w4)-2*c_py*(2*y_t2_dot-2*h_tp*theta_t2_dot-y_w3_dot-y_w4_dot)+f_2;
y_t2_ddot = y_t2_ddot/m_t;
end

== matlab function Lateral_control_of_HST/Differential equation of psi_t1 ==
  data: J_tz input; psi_t1_ddot output; k_sx input; psi_c input; psi_t1 input; d_s input; c_sx input; psi_c_dot input; psi_t1_dot input; k_px input; psi_w1 input; psi_w2 input; d_p input; c_px input; psi_w1_dot input; psi_w2_dot input; k_py input; b input; y_w1 input; y_w2 input; c_py input; y_w1_dot input; y_w2_dot input
function psi_t1_ddot = fcn(J_tz,k_sx,psi_c,psi_t1,d_s,c_sx,psi_c_dot,psi_t1_dot,k_px,psi_w1,psi_w2,d_p,c_px,psi_w1_dot,psi_w2_dot,k_py,b,y_w1,y_w2,c_py,y_w1_dot,y_w2_dot)
psi_t1_ddot = 0;
psi_t1_ddot = 2*k_sx*(psi_c-psi_t1)*d_s^2+2*c_sx*(psi_c_dot-psi_t1_dot)*d_s^2-2*k_px*(2*psi_t1-psi_w1-psi_w2)*d_p^2-2*c_px*(2*psi_t1_dot-psi_w1_dot-psi_w2_dot)*d_p^2-2*k_py*b*(2*b*psi_t1-y_w1+y_w2)-2*c_py*b*(2*b*psi_t1_dot-y_w1_dot+y_w2_dot);
psi_t1_ddot = psi_t1_ddot/J_tz;
end

== matlab function Lateral_control_of_HST/Differential equation of psi_t2 ==
  data: J_tz input; psi_t2_ddot output; k_sx input; psi_c input; psi_t2 input; d_s input; c_sx input; psi_c_dot input; psi_t2_dot input; k_px input; psi_w3 input; psi_w4 input; d_p input; c_px input; psi_w3_dot input; psi_w4_dot input; k_py input; b input; y_w3 input; y_w4 input; c_py input; y_w3_dot input; y_w4_dot input
function psi_t2_ddot = fcn(J_tz,k_sx,psi_c,psi_t2,d_s,c_sx,psi_c_dot,psi_t2_dot,k_px,psi_w3,psi_w4,d_p,c_px,psi_w3_dot,psi_w4_dot,k_py,b,y_w3,y_w4,c_py,y_w3_dot,y_w4_dot)
psi_t2_ddot = 0;
psi_t2_ddot = 2*k_sx*(psi_c-psi_t2)*d_s^2+2*c_sx*(psi_c_dot-psi_t2_dot)*d_s^2-2*k_px*(2*psi_t2-psi_w3-psi_w4)*d_p^2-2*c_px*(2*psi_t2_dot-psi_w3_dot-psi_w4_dot)*d_p^2-2*k_py*b*(2*b*psi_t2-y_w3+y_w4)-2*c_py*b*(2*b*psi_t2_dot-y_w3_dot+y_w4_dot);
psi_t2_ddot = psi_t2_ddot/J_tz;
end

== matlab function Lateral_control_of_HST/Differential equation of theta_t1 ==
  data: J_tx input; theta_t1_ddot output; k_sy input; h_ts input; y_c input; l input; psi_c input; h_cs input; theta_c input; y_t1 input; theta_t1 input; c_sy input; y_c_dot input; psi_c_dot input; theta_c_dot input; y_t1_dot input; theta_t1_dot input; k_sz input; d_s input; c_sz input; k_py input; h_tp input; y_w1 input; y_w2 input; c_py input; y_w1_dot input; y_w2_dot input; k_pz input; d_p input; c_pz input; f_1 input
function theta_t1_ddot = fcn(J_tx,k_sy,h_ts,y_c,l,psi_c,h_cs,theta_c,y_t1,theta_t1,c_sy,y_c_dot,psi_c_dot,theta_c_dot,y_t1_dot,theta_t1_dot,k_sz,d_s,c_sz,k_py,h_tp,y_w1,y_w2,c_py,y_w1_dot,y_w2_dot,k_pz,d_p,c_pz,f_1)
theta_t1_ddot = 0;
theta_t1_ddot = 2*k_sy*h_ts*(y_c+l*psi_c-h_cs*theta_c-y_t1-h_ts*theta_t1)+2*c_sy*h_ts*(y_c_dot+l*psi_c_dot-h_cs*theta_c_dot-y_t1_dot-h_ts*theta_t1_dot)+2*k_sz*(theta_c-theta_t1)*d_s^2+2*c_sz*(theta_c_dot-theta_t1_dot)*d_s^2+2*k_py*h_tp*(2*y_t1-2*h_tp*theta_t1-y_w1-y_w2)+2*c_py*h_tp*(2*y_t1_dot-2*h_tp*theta_t1_dot-y_w1_dot-y_w2_dot)-4*k_pz*d_p^2*theta_t1-4*c_pz*d_p^2*theta_t1_dot+f_1*h_ts;
theta_t1_ddot = theta_t1_ddot/J_tx;
end

== matlab function Lateral_control_of_HST/Differential equation of theta_t2 ==
  data: J_tx input; theta_t2_ddot output; k_sy input; h_ts input; y_c input; l input; psi_c input; h_cs input; theta_c input; y_t2 input; theta_t2 input; c_sy input; y_c_dot input; psi_c_dot input; theta_c_dot input; y_t2_dot input; theta_t2_dot input; k_sz input; d_s input; c_sz input; k_py input; h_tp input; y_w3 input; y_w4 input; c_py input; y_w3_dot input; y_w4_dot input; k_pz input; d_p input; c_pz input; f_2 input
function theta_t2_ddot = fcn(J_tx,k_sy,h_ts,y_c,l,psi_c,h_cs,theta_c,y_t2,theta_t2,c_sy,y_c_dot,psi_c_dot,theta_c_dot,y_t2_dot,theta_t2_dot,k_sz,d_s,c_sz,k_py,h_tp,y_w3,y_w4,c_py,y_w3_dot,y_w4_dot,k_pz,d_p,c_pz,f_2)
theta_t2_ddot =0;
theta_t2_ddot = 2*k_sy*h_ts*(y_c-l*psi_c-h_cs*theta_c-y_t2-h_ts*theta_t2)+2*c_sy*h_ts*(y_c_dot-l*psi_c_dot-h_cs*theta_c_dot-y_t2_dot-h_ts*theta_t2_dot)+2*k_sz*(theta_c-theta_t2)*d_s^2+2*c_sz*(theta_c_dot-theta_t2_dot)*d_s^2+2*k_py*h_tp*(2*y_t2-2*h_tp*theta_t2-y_w3-y_w4)+2*c_py*h_tp*(2*y_t2_dot-2*h_tp*theta_t2_dot-y_w3_dot-y_w4_dot)-4*k_pz*d_p^2*theta_t2-4*c_pz*d_p^2*theta_t2_dot+f_2*h_ts;
theta_t2_ddot = theta_t2_ddot/J_tx;
end

== matlab function Lateral_control_of_HST/Differential equation of y_w1 ==
  data: m_w input; y_w1_ddot output; k_py input; y_t1 input; b input; psi_t1 input; h_tp input; theta_t1 input; y_w1 input; c_py input; y_t1_dot input; psi_t1_dot input; theta_t1_dot input; y_w1_dot input; f_22 input; V input; sigma input; r_0 input; a input; y_a1_dot input; theta_cl1_dot input; psi_w1 input; K_gy input; y_a1 input; theta_cl1 input
function y_w1_ddot = fcn(m_w,k_py,y_t1,b,psi_t1,h_tp,theta_t1,y_w1,c_py,y_t1_dot,psi_t1_dot,theta_t1_dot,y_w1_dot,f_22,V,sigma,r_0,a,y_a1_dot,theta_cl1_dot,psi_w1,K_gy,y_a1,theta_cl1)
y_w1_ddot = 0;
y_w1_ddot = 2*k_py*(y_t1+b*psi_t1-h_tp*theta_t1-y_w1)+2*c_py*(y_t1_dot+b*psi_t1_dot-h_tp*theta_t1_dot-y_w1_dot)-2*f_22*(y_w1_dot/V-psi_w1)-K_gy*(y_w1-y_a1-r_0*theta_cl1);
y_w1_ddot = y_w1_ddot/m_w;
end

== matlab function Lateral_control_of_HST/Differential equation of y_w2 ==
  data: m_w input; y_w2_ddot output; k_py input; y_t1 input; b input; psi_t1 input; h_tp input; theta_t1 input; y_w2 input; c_py input; y_t1_dot input; psi_t1_dot input; theta_t1_dot input; y_w2_dot input; f_22 input; V input; sigma input; r_0 input; a input; y_a2_dot input; theta_cl2_dot input; psi_w2 input; K_gy input; y_a2 input; theta_cl2 input
function y_w2_ddot = fcn(m_w,k_py,y_t1,b,psi_t1,h_tp,theta_t1,y_w2,c_py,y_t1_dot,psi_t1_dot,theta_t1_dot,y_w2_dot,f_22,V,sigma,r_0,a,y_a2_dot,theta_cl2_dot,psi_w2,K_gy,y_a2,theta_cl2)
y_w2_ddot = 0;
y_w2_ddot = 2*k_py*(y_t1-b*psi_t1-h_tp*theta_t1-y_w2)+2*c_py*(y_t1_dot-b*psi_t1_dot-h_tp*theta_t1_dot-y_w2_dot)-2*f_22*(y_w2_dot/V-psi_w2)-K_gy*(y_w2-y_a2-r_0*theta_cl2);
y_w2_ddot = y_w2_ddot/m_w;
end

== matlab function Lateral_control_of_HST/Differential equation of psi_c ==
  data: J_cz input; psi_c_ddot output; k_sx input; psi_c input; psi_c_dot input; psi_t1 input; psi_t2 input; d_s input; c_sx input; psi_t1_dot input; psi_t2_dot input; k_sy input; l input; y_t1 input; y_t1_dot input; y_t2 input; y_t2_dot input; h_ts input; theta_t1 input; theta_t1_dot input; theta_t2 input; theta_t2_dot input; c_sy input; f_1 input; f_2 input
function psi_c_ddot = fcn(J_cz,k_sx,psi_c,psi_c_dot,psi_t1,psi_t2,d_s,c_sx,psi_t1_dot,psi_t2_dot,k_sy,l,y_t1,y_t1_dot,y_t2,y_t2_dot,h_ts,theta_t1,theta_t1_dot,theta_t2,theta_t2_dot,c_sy,f_1,f_2)
psi_c_ddot = 0;
psi_c_ddot = -2*k_sx*(2*psi_c-psi_t1-psi_t2)*d_s^2-2*c_sx*(2*psi_c_dot-psi_t1_dot-psi_t2_dot)*d_s^2-2*k_sy*(2*l*psi_c-y_t1+y_t2-h_ts*theta_t1+h_ts*theta_t2)*l-2*c_sy*(2*l*psi_c_dot-y_t1_dot+y_t2_dot-h_ts*theta_t1_dot+h_ts*theta_t2_dot)*l-(f_1-f_2)*l;
psi_c_ddot=psi_c_ddot/J_cz;
end

== matlab function Lateral_control_of_HST/Differential equation of y_w3 ==
  data: m_w input; y_w3_ddot output; k_py input; y_t2 input; b input; psi_t2 input; h_tp input; theta_t2 input; y_w3 input; c_py input; y_t2_dot input; psi_t2_dot input; theta_t2_dot input; y_w3_dot input; f_22 input; V input; sigma input; r_0 input; a input; y_a3_dot input; theta_cl3_dot input; psi_w3 input; K_gy input; y_a3 input; theta_cl3 input
function y_w3_ddot = fcn(m_w,k_py,y_t2,b,psi_t2,h_tp,theta_t2,y_w3,c_py,y_t2_dot,psi_t2_dot,theta_t2_dot,y_w3_dot,f_22,V,sigma,r_0,a,y_a3_dot,theta_cl3_dot,psi_w3,K_gy,y_a3,theta_cl3)
y_w3_ddot = 0;
y_w3_ddot = 2*k_py*(y_t2+b*psi_t2-h_tp*theta_t2-y_w3)+2*c_py*(y_t2_dot+b*psi_t2_dot-h_tp*theta_t2_dot-y_w3_dot)-2*f_22*(y_w3_dot/V-psi_w3)-K_gy*(y_w3-y_a3-r_0*theta_cl3);
y_w3_ddot = y_w3_ddot/m_w;
end

== matlab function Lateral_control_of_HST/Differential equation of y_w4 ==
  data: m_w input; y_w4_ddot output; k_py input; y_t2 input; b input; psi_t2 input; h_tp input; theta_t2 input; y_w4 input; c_py input; y_t2_dot input; psi_t2_dot input; theta_t2_dot input; y_w4_dot input; f_22 input; V input; sigma input; r_0 input; a input; y_a4_dot input; theta_cl4_dot input; psi_w4 input; K_gy input; y_a4 input; theta_cl4 input
function y_w4_ddot = fcn(m_w,k_py,y_t2,b,psi_t2,h_tp,theta_t2,y_w4,c_py,y_t2_dot,psi_t2_dot,theta_t2_dot,y_w4_dot,f_22,V,sigma,r_0,a,y_a4_dot,theta_cl4_dot,psi_w4,K_gy,y_a4,theta_cl4)
y_w4_ddot = 0;
y_w4_ddot = 2*k_py*(y_t2-b*psi_t2-h_tp*theta_t2-y_w4)+2*c_py*(y_t2_dot-b*psi_t2_dot-h_tp*theta_t2_dot-y_w4_dot)-2*f_22*(y_w4_dot/V-psi_w4)-K_gy*(y_w4-y_a4-r_0*theta_cl4);
y_w4_ddot = y_w4_ddot/m_w;
end

== matlab function Lateral_control_of_HST/Differential equation of psi_w1  ==
  data: J_wz input; psi_w1_ddot output; k_px input; psi_t1 input; psi_w1 input; d_p input; c_px input; psi_t1_dot input; psi_w1_dot input; f_11 input; lambda_e input; y_w1 input; y_a1 input; theta_cl1 input; V input; K_gpsi input; a input; r_0 input
function psi_w1_ddot = fcn(J_wz,k_px,psi_t1,psi_w1,d_p,c_px,psi_t1_dot,psi_w1_dot,f_11,lambda_e,y_w1,y_a1,theta_cl1,V,K_gpsi,a,r_0)
psi_w1_ddot = 0;
psi_w1_ddot = 2*k_px*(psi_t1-psi_w1)*d_p^2+2*c_px*(psi_t1_dot-psi_w1_dot)*d_p^2-2*f_11*(lambda_e*a*y_w1/r_0+a^2*psi_w1_dot/V)+K_gpsi*psi_w1+2*f_11*lambda_e*a*(y_a1+r_0*theta_cl1)/r_0;
psi_w1_ddot = psi_w1_ddot/J_wz;
end

== matlab function Lateral_control_of_HST/Differential equation of psi_w2 ==
  data: J_wz input; psi_w2_ddot output; k_px input; psi_t1 input; psi_w2 input; d_p input; c_px input; psi_t1_dot input; psi_w2_dot input; f_11 input; lambda_e input; y_w2 input; y_a2 input; theta_cl2 input; V input; K_gpsi input; a input; r_0 input
function psi_w2_ddot = fcn(J_wz,k_px,psi_t1,psi_w2,d_p,c_px,psi_t1_dot,psi_w2_dot,f_11,lambda_e,y_w2,y_a2,theta_cl2,V,K_gpsi,a,r_0)
psi_w2_ddot = 0;
psi_w2_ddot = 2*k_px*(psi_t1-psi_w2)*d_p^2+2*c_px*(psi_t1_dot-psi_w2_dot)*d_p^2-2*f_11*(lambda_e*a*(y_w2-y_a2-r_0*theta_cl2)/r_0+a^2*psi_w2_dot/V)+K_gpsi*psi_w2;
psi_w2_ddot = psi_w2_ddot/J_wz;
end

== matlab function Lateral_control_of_HST/Differential equation of psi_w3 ==
  data: J_wz input; psi_w3_ddot output; k_px input; psi_t2 input; psi_w3 input; d_p input; c_px input; psi_t2_dot input; psi_w3_dot input; f_11 input; lambda_e input; y_w3 input; y_a3 input; theta_cl3 input; V input; K_gpsi input; a input; r_0 input
function psi_w3_ddot = fcn(J_wz,k_px,psi_t2,psi_w3,d_p,c_px,psi_t2_dot,psi_w3_dot,f_11,lambda_e,y_w3,y_a3,theta_cl3,V,K_gpsi,a,r_0)
psi_w3_ddot = 0;
psi_w3_ddot = 2*k_px*(psi_t2-psi_w3)*d_p^2+2*c_px*(psi_t2_dot-psi_w3_dot)*d_p^2-2*f_11*(lambda_e*a*(y_w3-y_a3-r_0*theta_cl3)/r_0+a^2*psi_w3_dot/V)+K_gpsi*psi_w3;
psi_w3_ddot = psi_w3_ddot/J_wz;
end

== matlab function Lateral_control_of_HST/Differential equation of psi_w4 ==
  data: J_wz input; psi_w4_ddot output; k_px input; psi_t2 input; psi_w4 input; d_p input; c_px input; psi_t2_dot input; psi_w4_dot input; f_11 input; lambda_e input; y_w4 input; y_a4 input; theta_cl4 input; V input; K_gpsi input; a input; r_0 input
function psi_w4_ddot = fcn(J_wz,k_px,psi_t2,psi_w4,d_p,c_px,psi_t2_dot,psi_w4_dot,f_11,lambda_e,y_w4,y_a4,theta_cl4,V,K_gpsi,a,r_0)
psi_w4_ddot = 0;
psi_w4_ddot = 2*k_px*(psi_t2-psi_w4)*d_p^2+2*c_px*(psi_t2_dot-psi_w4_dot)*d_p^2-2*f_11*(lambda_e*a*(y_w4-y_a4-r_0*theta_cl4)/r_0+a^2*psi_w4_dot/V)+K_gpsi*psi_w4;
psi_w4_ddot = psi_w4_ddot/J_wz;
end

== matlab function Lateral_control_of_HST/Subsystem3/MATLAB Function ==
  data: t input; y output; d_hat input
function y = fcn(t,d_hat)
if(t<2)
y = 0;
else
    y=d_hat;
end

== matlab function Lateral_control_of_HST/F_wind ==
  settings: updateMethod=DISCRETE  sampleTime=0.01
  data: t input; F_side output; v_train input; w_mean input; M_roll output; w_c output
function [F_side, M_roll ,w_c] = turbulent_wind_model(t, v_train, w_mean)

persistent initialized L_veh dt_coarse t_coarse w_prime w_c_prime u_rel0 tau
if isempty(initialized)
    % 基本参数
    L_veh = 25.0;      
    dt_coarse = 0.05;    
    t_coarse = 0:dt_coarse:600; 

    h0 = 0.07;         
    h_ref = 4.0;       
    a1 = log(h_ref / h0);
    a2 = 1 - (5 / 10^5) * (log10(h0/0.05) + 2)^7;
    I_z = a2 / a1;
    % 计算湍流特性
    sigma_w = I_z * w_mean;              % 风速标准差 (式5)
    L_u = 50 * (h_ref^0.35)/(h0^0.063);  % 湍流积分尺度 (式7)
    u_rel0 = sqrt(v_train^2 + w_mean^2); % 初始相对风速

    % 生成原始湍流序列 (随机相位法)
    rng(0); % 固定随机种子
    N = length(t_coarse);
    w_prime = zeros(1, N);

    % Cooper谱参数 (式12)
    L_u_prime = L_u * sqrt((w_mean/u_rel0)^2 + 4*(0.42)^2*(w_mean/u_rel0)^2);

    % 生成频域分量
    f_min = 0.001; f_max = 10; df = 0.001;
    f = f_min:df:f_max;
    phi = 2*pi*rand(size(f)); % 随机相位

    for i = 1:N
        t_val = t_coarse(i);
        w_prime(i) = 0;
        for k = 1:length(f)
            % Cooper谱计算 (式12)
            f_dim = f(k) * L_u_prime / u_rel0;
            term1 = 4 * f_dim / (1 + 70.8*f_dim^2)^(5/6);
            term2 = (w_mean/u_rel0)^2 + ...
                   (1 - (w_mean/u_rel0)^2)*...
                   (0.5 + 94.4*f_dim^2)/(1 + 70.8*f_dim^2);
            S_w = (sigma_w^2 / f(k)) * term1 * term2;

            % 傅里叶分量叠加
            amp = sqrt(2 * S_w * df);
            w_prime(i) = w_prime(i) + amp * cos(2*pi*f(k)*t_val + phi(k));
        end
    end

    % 导纳函数修正 (递归指数滤波)
    tau = L_veh / u_rel0;  % 时间常数
    w_c_prime = zeros(1, N);
    w_c_prime(1) = w_prime(1);

    for i = 2:N
        alpha = exp(-dt_coarse/tau);
        w_c_prime(i) = alpha * w_c_prime(i-1) + (1-alpha) * w_prime(i);
    end

    % 空间平均滤波 (论文2.3节)
    window_size = max(1, round(L_veh/(v_train*dt_coarse)));
    w_c_prime = movmean(w_c_prime, window_size);

    initialized = true;
end

% ====== 实时计算部分 (每0.001s执行) ======
% 1. 获取当前修正风速 (线性插值)
idx = floor(t/dt_coarse) + 1;
if idx < length(t_coarse)
    frac = (t - t_coarse(idx)) / dt_coarse;
    w_c = w_mean + w_c_prime(idx) + frac*(w_c_prime(idx+1) - w_c_prime(idx));
else
    w_c = w_mean + w_c_prime(end); % 超出范围使用末值
end

% 2. 计算修正气动参数 (式24-25)
u_rel = sqrt(v_train^2 + w_c^2);   % 当前相对风速
beta_c = atan(w_c / v_train);      % 修正偏航角 (rad)

% 3. 气动系数查询 (替换为实际数据)
beta_deg = rad2deg(beta_c);
[CF, CM] = aerodynamic_coefficients(beta_deg);

% 4. 计算气动力/力矩 (式22-23)
rho = 1.225; A = 10; h = 3;
if(t>0)
        F_side = 0.5 * rho * A * CF * u_rel^2; 
        M_roll = 0.5 * rho * A * h * CM * u_rel^2;
else
    F_side = 0;
    M_roll = 0;
end
end
function [CF, CM] = aerodynamic_coefficients(beta_deg)
    beta_data = [0, 5.73, 8.59, 11.46, 14.32, 17.19, 20.05, 22.92, 25.79];
    CF_data   = [0, 0.51, 0.78, 1.11, 1.38, 1.72 ,2.15, 2.52, 2.86];                                                                                                                             
    CM_data   = [0, -0.083,-0.125,-0.167,-0.208,-0.25,-0.291,-0.33,-0.375];    
    query_val = min(max(beta_deg, 0), 25.79);
    CF = interp1(beta_data, CF_data, query_val, 'linear');
    CM = interp1(beta_data, CM_data, query_val, 'linear');
end

== matlab function Lateral_control_of_HST/MATLAB Function8 ==
  data: t input; y output
function y = fcn(t)
if(t<5)
    y = -30;
elseif(t<33)
    y = 20;
else
    y = 40;
end

== matlab function Lateral_control_of_HST/MATLAB Function9 ==
  data: t input; y output
function y = fcn(t)
if(t<10)
    y = -100;
elseif(t<30)
    y = 300;
else
    y = 500;
end

== matlab function Lateral_control_of_HST/MATLAB Function16 ==
  data: t input; y output
function y = fcn(t)
if(t<10)
    y = 0;
elseif(t<20)
    y = 20;
else
    y = 40;
end

== matlab function Lateral_control_of_HST/MATLAB Function10 ==
  data: i input; y output; x input
function y = fcn(i,x)
A = 32*6+918*6*i-244*6*i*i;
z = tanh(100+(0.58+0.3*i)*sign(x));
y = A*z;

== matlab function Lateral_control_of_HST/MATLAB Function5 ==
  data: sigma_c input; uc output; sigma_dot_c input
function uc = fcn(sigma_c, sigma_dot_c)
    numerator = sigma_dot_c + 20 * abs(sigma_c)^0.5 * sign(sigma_c);
    denominator = abs(sigma_dot_c) + 20 * abs(sigma_c)^0.5;
    if denominator == 0
        uc = 0;
    else
        uc = -300*(numerator/denominator);%257
    end

== matlab function Lateral_control_of_HST/MATLAB Function6 ==
  data: sigma_t input; ut output; sigma_dot_t input
function ut = fcn(sigma_t, sigma_dot_t)
    numerator = sigma_dot_t + 20 * abs(sigma_t)^0.5 * sign(sigma_t);
    denominator = abs(sigma_dot_t) + 20 * abs(sigma_t)^0.5;
    if denominator == 0
        ut = 0;
    else
        ut = -100*(numerator/denominator);
    end
end

== matlab function Lateral_control_of_HST/MATLAB Function7 ==
  data: i input; y output; x input
function y = fcn(i,x)
A = 32*6+918*6*i-244*6*i*i;
z = tanh(100+(0.58+0.3*i)*sign(x));
y = A*z;

== matlab function Lateral_control_of_HST/Differential equation of y_c ==
  data: m_c input; y_c_ddot output; k_sy input; y_c input; h_cs input; theta_c input; y_t1 input; y_t2 input; h_ts input; theta_t1 input; theta_t2 input; c_sy input; y_c_dot input; theta_c_dot input; y_t1_dot input; y_t2_dot input; theta_t1_dot input; theta_t2_dot input; f_1 input; f_2 input; F_wind input; y1 output; y2 output; y3 output; y4 output; y5 output; y6 output
function [y_c_ddot,y1,y2,y3,y4,y5,y6] = fcn(m_c, k_sy, y_c, h_cs, theta_c, y_t1, y_t2, h_ts, theta_t1, theta_t2, c_sy, y_c_dot, theta_c_dot, y_t1_dot, y_t2_dot, theta_t1_dot, theta_t2_dot, f_1, f_2,F_wind)
y_c_ddot = 0;
y_c_ddot = -2*k_sy*(2*y_c - 2*h_cs*theta_c - y_t1 - y_t2 - h_ts*theta_t1 - h_ts*theta_t2) - 2*c_sy*(2*y_c_dot - 2*h_cs*theta_c_dot - y_t1_dot - y_t2_dot - h_ts*theta_t1_dot - h_ts*theta_t2_dot) - (f_1 + f_2) + F_wind;
y1 = -2*k_sy*(2*y_c - 2*h_cs*theta_c) - 2*c_sy*(2*y_c_dot - 2*h_cs*theta_c_dot);
y2 = -2*k_sy*(- y_t1 - y_t2 - h_ts*theta_t1 - h_ts*theta_t2)- 2*c_sy*(- y_t1_dot - y_t2_dot - h_ts*theta_t1_dot - h_ts*theta_t2_dot);
y5 = F_wind;
y4 = -2*k_sy*(2*y_c - 2*h_cs*theta_c - y_t1 - y_t2 - h_ts*theta_t1 - h_ts*theta_t2) - 2*c_sy*(2*y_c_dot - 2*h_cs*theta_c_dot - y_t1_dot - y_t2_dot - h_ts*theta_t1_dot - h_ts*theta_t2_dot) + F_wind;
y3 = -(f_1 + f_2);
y6 = -2*k_sy*(2*y_c - 2*h_cs*theta_c - y_t1 - y_t2 - h_ts*theta_t1 - h_ts*theta_t2) - 2*c_sy*(2*y_c_dot - 2*h_cs*theta_c_dot - y_t1_dot - y_t2_dot - h_ts*theta_t1_dot - h_ts*theta_t2_dot) - (f_1 + f_2) + F_wind;
y_c_ddot = y_c_ddot / m_c;
end

== matlab function Lateral_control_of_HST/Differential equation of theta_c ==
  data: J_cx input; theta_c_ddot output; k_sy input; y_c input; h_cs input; theta_c input; y_t1 input; y_t2 input; h_ts input; theta_t1 input; theta_t2 input; c_sy input; y_c_dot input; theta_c_dot input; y_t1_dot input; y_t2_dot input; theta_t1_dot input; theta_t2_dot input; k_sz input; d_s input; c_sz input; f_1 input; f_2 input; F_wind input; y1 output; y2 output; y3 output; y4 output; y5 output; y6 output
function [theta_c_ddot,y1,y2,y3,y4,y5,y6] = fcn(J_cx,k_sy,y_c,h_cs,theta_c,y_t1,y_t2,h_ts,theta_t1,theta_t2,c_sy,y_c_dot,theta_c_dot,y_t1_dot,y_t2_dot,theta_t1_dot,theta_t2_dot,k_sz,d_s,c_sz,f_1,f_2,F_wind)
theta_c_ddot = 0;
theta_c_ddot = 2*k_sy*h_cs*(2*y_c-2*h_cs*theta_c-y_t1-y_t2-h_ts*theta_t1-h_ts*theta_t2)+2*c_sy*h_cs*(2*y_c_dot-2*h_cs*theta_c_dot-y_t1_dot-y_t2_dot-h_ts*theta_t1_dot-h_ts*theta_t2_dot)-2*k_sz*(2*theta_c-theta_t1-theta_t2)*d_s^2-2*c_sz*(2*theta_c_dot-theta_t1_dot-theta_t2_dot)*d_s^2 +(f_1+f_2)*h_cs + 0.1*F_wind;
y1 = 2*k_sy*h_cs*(2*y_c-2*h_cs*theta_c-y_t1-y_t2-h_ts*theta_t1-h_ts*theta_t2);
y2 = 2*c_sy*h_cs*(2*y_c_dot-2*h_cs*theta_c_dot-y_t1_dot-y_t2_dot-h_ts*theta_t1_dot-h_ts*theta_t2_dot);
y3 = -2*k_sz*(2*theta_c-theta_t1-theta_t2)*d_s^2-2*c_sz*(2*theta_c_dot-theta_t1_dot-theta_t2_dot)*d_s^2;
y4 = +(f_1+f_2)*h_cs;
y5 =  +0.1*F_wind;
y6 = 2*k_sy*h_cs*(2*y_c-2*h_cs*theta_c-y_t1-y_t2-h_ts*theta_t1-h_ts*theta_t2)+2*c_sy*h_cs*(2*y_c_dot-2*h_cs*theta_c_dot-y_t1_dot-y_t2_dot-h_ts*theta_t1_dot-h_ts*theta_t2_dot)-2*k_sz*(2*theta_c-theta_t1-theta_t2)*d_s^2-2*c_sz*(2*theta_c_dot-theta_t1_dot-theta_t2_dot)*d_s^2 +(f_1+f_2)*h_cs + 0.1*F_wind;
theta_c_ddot = theta_c_ddot/J_cx;
end
